simulink model "EcoSIM3_P2_C2"  (R2014b)
settings: Solver=ode1  SolverMode=SingleTasking  StartTime=0.0  StopTime=inf  FixedStep=0.01  RelTol=1e-3
PostLoadFcn:
  | %, if any(exist('dsrtsu_mdlpostloadfcn', 'file') == [2, 3, 6]), try dsrtsu_mdlpostloadfcn('Execute', bdroot); catch fprintf('Error in PostLoadFcn (dsrtsu_mdlpostloadfcn) for model "%s":\n %s\n', bdroot, lasterr); end, end,
InitFcn:
  | tic
  | %Startup_EcoSIM
values from neighbouring files (symbols this model uses):
  EngPwr = [0 5	10	15	20	25	30	35	40	45	50	55	60	65	70	75	80	85	90	95	100	105	110	115]    [Series_Maps.m]
  EngSpd = [0 477.4645 954.929 1909.858 2864.787 3819.716 4774.645 5729.574 6684.503]    [Series_Maps.m]
  EngTrq = [0	0	0	0	0	0	0	0	0	0	0	0	0	0	0	0	0	0	0	0	0	0	0	0 ... (first row only)    [Series_Maps.m]
  Power = [0 5 10 15 20 25 30]    [Series_Maps.m]
  Torque = [-50,-40,-30,-25,-20,-15,-10,-8,-6,-4,-2,0]    [Series_Maps.m]
undefined symbols (not defined in the file or in its folder): canChannel, Controls, DriveCycles, Driver, EM_EFF_MAP, EM_PwrLoss_MAP, Glbl, Plants, Veh_Dynamics
libraries: canmsglib x100, canlib x87, fl_lib x78, simulink x59, nesl_utility x40, sdl_lib x17, dspsigops x5, dspswit3 x3, dspstat3 x2, commnoisgen2 x1, dspfdesign x1
(part 15 of 15)

== stateflow chart EcoSIM3_P2_C2/Powertrain/BAS Motor/Soft ECU/Algorithm/BAS_Stateflow/BAS SoftECU ==
  note: Mode Request is similar to Inverter Enable / Disable
  state StartupShutdownSequence [group]
    state StartState
      during: Commanded_Torque = 0;
      %Loading EEPROM Parameters & carrying out POST (Power On Self Tests)
    state Standby
      % Entry point into Inverter
      % State Machine
    state Startup_Sequence
      state Inverter_Wait
        entry: FaultState=0;
        during: Commanded_Torque =0;
      state Inverter_Ready
        during: Commanded_Torque =0;
        entry: InverterStatusMode = 1;
        during: InverterStatusMode = 1;
      Inverter_Wait -> Inverter_Ready : [ModeRequest >= 1]
    state NormalOperation
      exit:Commanded_Torque=0;
      state Speed_Control_Mode
        state ValidSpeed
          entry: Commanded_Speed=Speed_Command;
          during: Commanded_Speed=Speed_Command;
        (default) -> StartupShutdownSequence.NormalOperation.Speed_Control_Mode.ValidSpeed
      state Torque_Control_Mode
        state SpeedGreaterThanMaxSpeed
          entry: Commanded_Torque=0;
          during: Commanded_Torque = 0;
        state ValidSpeed
          entry: Commanded_Torque=Torque_Command;
          during: Commanded_Torque=Torque_Command;
        state SpeedGreaterThanMaxSpeed1 [commented out]
          entry: Commanded_Torque=0;
        (default) -> (junction 53)
        (junction 53) -> SpeedGreaterThanMaxSpeed [order 1] : [abs (MotorSpeed) > MotorMaxSpeed]
        (junction 53) -> (junction 60) [order 2]
        SpeedGreaterThanMaxSpeed -> (junction 60) : [abs (MotorSpeed) <= MotorMaxSpeed]
        (junction 60) -> StartupShutdownSequence.NormalOperation.Torque_Control_Mode.ValidSpeed
        StartupShutdownSequence.NormalOperation.Torque_Control_Mode.ValidSpeed -> SpeedGreaterThanMaxSpeed [commented out] : [abs (MotorSpeed) > MotorMaxSpeed]
        StartupShutdownSequence.NormalOperation.Torque_Control_Mode.ValidSpeed -> SpeedGreaterThanMaxSpeed1 [commented out] : [MotorSpeed<= 83*BeltRatio]
        SpeedGreaterThanMaxSpeed1 -> StartupShutdownSequence.NormalOperation.Torque_Control_Mode.ValidSpeed [commented out] : [MotorSpeed>84*BeltRatio]
      (default) -> (junction 101)
      (junction 101) -> Speed_Control_Mode [order 2] : [ModeRequest == 2]
      (junction 101) -> Torque_Control_Mode [order 1] : [ModeRequest == 1]
    state ShutdownInProcess
    state FaultState
      entry: FaultState = 1;
      during: FaultState = 1;
      % to exit this state, power must be cycled
    (default) -> Standby
    Standby -> StartState : [Power_up == 1 && ...
        | POST_Fault == 0 ]
    StartState -> FaultState [order 2] : [Power_up == 1 ...
        | &&POST_Fault == 1]
    StartState -> Inverter_Wait [order 1] : [Power_up == 1 ...
        | &&POST_Fault == 0]
    ShutdownInProcess -> Standby : [Power_up == 0]
    (junction 28) -> ShutdownInProcess [order 2] : [Power_up ==0]
    FaultState -> ShutdownInProcess : [Power_up == 0 ]
    Inverter_Ready -> NormalOperation : [MotorFault==0]
    (junction 28) -> FaultState [order 1] : [MotorFault ==1]
    NormalOperation -> (junction 28) : [MotorFault==1]
  data: Power_up input; MotorFault input; ModeRequest input; Commanded_Torque output; MotorMaxSpeed input; POST_Fault input; InverterStatusMode output; Torque_Command input; MotorSpeed input; FaultState output; BeltRatio input; Commanded_Speed output; Speed_Command input

== stateflow chart EcoSIM3_P2_C2/Powertrain/Electric Motor /Soft ECU/Algorithm/Startup_Shutdown/Startup-Shutdown ==
  state StartupShutdownSequence [group]
    state StartState
      entry: VSM_Mode = 0;
      during: Commanded_Torque = 0;
      %Loading EEPROM Parameters & carrying out POST (Power On Self Tests)
    state Standby
      % Entry point into Inverter
      % State Machine
    state Startup_Sequence
      state Inverter_Wait
        entry: VSM_Mode = 4;
        during: VSM_Mode = 4;
        during: Commanded_Torque =0;
        % Precharge_Bypasseed_EEPROM = 1
      state InverterEnableLockout
        entry: VSM_Mode = 5;
        during: VSM_Mode = 5;
        during: Commanded_Torque =0;
        entry: Inverter_Enable_Lockout = 1;
        during:Inverter_Enable_Lockout = 1;
      state Wait
      state MotorReady
        entry: Inverter_Enable_Lockout = 0;
        entry: Inverter_Status=1;
        during: Inverter_Enable_Lockout = 0;
      state MotorOnCommand
        entry: VSM_Mode=6;
      Inverter_Wait -> InverterEnableLockout : [KeySwMode == 0 && ...
          | IgnitionKeySw == 2]
      InverterEnableLockout -> Wait : [Inverter_Enable == 0]
      Wait -> MotorReady : after(0.05,sec)
      MotorReady -> MotorOnCommand : [InternalMotorError==0 && Inverter_Enable == 1]
    state ShutdownInProcess
      entry: VSM_Mode = 14;
      entry: Inverter_Enable_Lockout=1;
      entry: Inverter_Status=0;
      during: VSM_Mode = 14;
    state FaultState
      entry: VSM_Mode = 7;
      during: VSM_Mode = 7;
    (junction 28) -> Standby [order 2]
    Standby -> StartState : [Power_up == 1]
    (default) -> (junction 28)
    ShutdownInProcess -> Standby : [KeySwMode == 0 && ...
        | IgnitionKeySw == 0 ...
        | && Power_up == 0]
    StartState -> FaultState [order 2] : [POST_Fault == 1]
    StartState -> Inverter_Wait [order 1] : [Power_up ==1 && ...
        | ~InternalMotorError && POST_Fault == 0 ...
        | && batt_mainc_stat == 1 ]
    (junction 28) -> FaultState [order 1] : [InternalMotorError ==1]
    FaultState -> ShutdownInProcess : [(KeySwMode == 0 && ...
        | IgnitionKeySw == 0) ]
    MotorOnCommand -> ShutdownInProcess [order 1] : [ShutdownRequest ==1]
    MotorOnCommand -> FaultState [order 2] : [RUN_Fault==1]
  data: Power_up input; VSM_Mode output; InternalMotorError input; batt_mainc_stat input; Inverter_Enable input; IgnitionKeySw input; Inverter_Enable_Lockout output; RUN_Fault input; Commanded_Torque local; ShutdownRequest input; KeySwMode input; POST_Fault input; Inverter_Status output

== stateflow chart EcoSIM3_P2_C2/Powertrain/Electric Motor /Soft ECU/Algorithm/Normal Operation/Normal_Operation ==
  state NormalOperation
    entry: set_direction=Rotation_Direction;
    entry: ShutdownRequest=0;
    exit: Commanded_Torque=0;
    state SpeedGreaterThanMaxSpeed
      entry: Commanded_Torque=0;
    state ValidSpeed
      entry: Commanded_Torque=Torque_Command;
      during: Commanded_Torque=Torque_Command;
    (default) -> (junction 9)
    (junction 9) -> SpeedGreaterThanMaxSpeed [order 1] : [abs (Motor_Speed) > Motor_MaxSpeed]
    (junction 9) -> (junction 10) [order 2]
    SpeedGreaterThanMaxSpeed -> (junction 10) : [abs (Motor_Speed) <= Motor_MaxSpeed]
    (junction 10) -> ValidSpeed
    ValidSpeed -> SpeedGreaterThanMaxSpeed : [abs (Motor_Speed) > Motor_MaxSpeed]
  state Fault
    entry: RUN_Fault=1;
  state ShutdownRequest
    entry: ShutdownRequest=1;
  (default) -> NormalOperation
  NormalOperation -> Fault [order 1] : [ InternalMotorError ==1||batt_mainc_stat==0]
  NormalOperation -> ShutdownRequest [order 2] : [IgnitionKeySw==0||...
      | Inverter_Enable==0]
  ShutdownRequest -> NormalOperation : [IgnitionKeySw==2||...
      | Inverter_Enable==1]
  data: Motor_Speed input; InternalMotorError input; Rotation_Direction input; set_direction local; Commanded_Torque output; Torque_Command input; batt_mainc_stat input; Inverter_Enable input; IgnitionKeySw input; RUN_Fault output; Motor_MaxSpeed input; ShutdownRequest output

== stateflow chart EcoSIM3_P2_C2/GCM/ProcessMode/Chart ==
  state Entry
    entry: charge_mode_request=0;
    Relay_Charge=0;
    Relay_Vehicle=0;
  state FaultModeDecideLater
  state VehicleRunMode
    entry: charge_mode_request=0;
    Relay_Charge=1;
    Relay_Vehicle=1;
  state ChargingMode
    entry: charge_mode_request=1;
    Relay_Charge=1;
    Relay_Vehicle=0;
  (default) -> Entry
  VehicleRunMode -> Entry : [Key_State==0]
  ChargingMode -> Entry [order 1] : [Key_State==0]
  Entry -> VehicleRunMode [order 1] : [Key_State==1 && ...
      | GCM_Wakeup_charge==0]
  Entry -> FaultModeDecideLater [order 3] : [Key_State==1 && ...
      | GCM_Wakeup_charge ==1]
  Entry -> ChargingMode [order 2] : [Key_State ==0 && ...
      | GCM_Wakeup_charge==1]
  ChargingMode -> FaultModeDecideLater [order 2] : [Key_State==1]
  data: Key_State input; GCM_Wakeup_charge input; charge_mode_request output; Relay_Charge output; Relay_Vehicle output

== matlab function EcoSIM3_P2_C2/Supervisory Controller/Functional Safety1/Functional Safety Algorithm/Fault Management/Truth Table ==
  data: u input; y output
function y = fcn(u)

aVarTruthTableCondition_1 = false;
aVarTruthTableCondition_2 = false;


% Example condition 1

aVarTruthTableCondition_1 = logical(u >= 0);

% Example condition 2

aVarTruthTableCondition_2 = logical(u ^ 2 <= 1);

if (aVarTruthTableCondition_1 && aVarTruthTableCondition_2)
    aFcnTruthTableAction_1();
elseif (~aVarTruthTableCondition_1 && ~aVarTruthTableCondition_2)
    aFcnTruthTableAction_1();
else % Default
    aFcnTruthTableAction_2();
end

function aFcnTruthTableAction_1()

% Example action 1 called from D1 & D2 column in condition table

y = u;

function aFcnTruthTableAction_2()

% Example action 2 called from D3 column in condition table

y = 1 / u;

== stateflow chart EcoSIM3_P2_C2/Powertrain/Engine/Soft ECU/Algorithm/ECM SoftECU ==
  state Entry
    entry: Torque_Cmd=0;
  state PoweredUp
    entry: Torque_Cmd=0;
  state PoweredUp1
    entry: Torque_Cmd=Torque_Request;
    du: Torque_Cmd=Torque_Request;
  state PoweredUp2
    entry: Torque_Cmd=0;
  (default) -> Entry
  PoweredUp1 -> Entry [order 1] : [ECM_Powerup==0]
  Entry -> PoweredUp : [ECM_Powerup==1]
  PoweredUp1 -> PoweredUp [order 2] : [PCM_Wake==0 || ...
      | ISP_R ==0]
  PoweredUp -> PoweredUp1 : [PCM_Wake==1 &&...
      | ISP_R==1]
  PoweredUp1 -> PoweredUp2 [order 3] : [Engine_Speed>Max_Speed]
  PoweredUp2 -> PoweredUp1 : [Engine_Speed <(Max_Speed-10)]
  data: Engine_Speed input; ECM_Powerup input; Torque_Cmd output; Torque_Request input; PCM_Wake input; ISP_R input; Max_Speed input

== stateflow chart EcoSIM3_P2_C2/Supervisory Controller/Mode Operation/Limited EV/Temperature Limiting/Chart ==
  state EM
    entry: out=1
  state Normal
    entry: out=4;
  state Inverter
    entry: out=2
  state Battery
    entry: out=3
  Normal -> EM [order 1] : [EM>100]
  (default) -> Normal
  Normal -> Inverter [order 2] : [Inverter>70]
  Normal -> Battery [order 3] : [Battery>50]
  data: EM input; Inverter input; Battery input; out output

== stateflow chart EcoSIM3_P2_C2/Fault Insertion/ESS Triggers/Chart ==
  state init
    en: output = 40;
  state stage1
    en: output = 56;
  state stage2
    en: output = 66;
  state stage3
    en: output = 40;
  (default) -> init
  init -> stage1 : [in == 1]
  stage1 -> stage2 : after(20, sec)
  stage2 -> stage3 : after(20, sec)
  data: in input; output output

== stateflow chart EcoSIM3_P2_C2/Supervisory Controller/Mode Operation/Shutdown/EM Handshake ==
  state Entry
  state DisableInverter
    entry: Inverter_Enable=0;
    during: Inverter_Enable=0;
  (default) -> Entry
  Entry -> DisableInverter : [Inverter_Enable_Lockout==1]
  data: Inverter_Enable_Lockout input; Inverter_Enable output

== stateflow chart EcoSIM3_P2_C2/Supervisory Controller/Mode Operation/Shutdown/Shutdown/ESS Handshake ==
  note: The ESS handshake ensures that the hsc_bcm_enable signal commands is sent by the supervisory only when the bcm is in the appropriate readiness state
  state WaitforBCMReady1
  state Disable
    entry: hsc_bcm_enable=0;
    during: hsc_bcm_enable=0;
  state OpenContactors
    entry:hsc_bcm_mainc_close=0;
    entry: hsc_bcm_leakage_ena=1;
    during:hsc_bcm_mainc_close=0;
    during:hsc_bcm_enable=0;
  Disable -> WaitforBCMReady1 : [bcm_ready==0]
  OpenContactors -> Disable : [bcm_mainc_stat==0]
  (default) -> OpenContactors
  data: bcm_ready input double; bcm_cpwr_cmd input double; bcm_cpwr_mon input double; hsc_bcm_enable output double; hsc_bcm_mainc_close output double; hsc_bcm_leakage_ena output; bcm_veh_mon input; Veh_Start input double; bcm_mainc_stat input

== stateflow chart EcoSIM3_P2_C2/Supervisory Controller/Mode Operation/Startup/BAS Start up/BAS Handshake ==
  state Entry
    entry: BAS_Mode_Request=0;
  state EnableBASInverter
    entry: BAS_Mode_Request=1;
  (default) -> Entry
  Entry -> EnableBASInverter : [BAS_Fault_Status==0 ...
      | && bcm_mainc_stat==1]
  data: BAS_Fault_Status input; bcm_mainc_stat input; BAS_Mode_Request output

== stateflow chart EcoSIM3_P2_C2/Supervisory Controller/Mode Operation/Startup/Battery Start Up /ESS Handshake ==
  note: The ESS handshake ensures that the hsc_bcm_enable signal commands is sent by the supervisory only when the bcm is in the appropriate readiness state
  state Entry
    entry: hsc_bcm_enable=0;
    en: hsc_bcm_leakage_ena=1;
    en: hsc_bcm_mainc_close=0;
  state WaitforBCMReady
  state Enable
    entry: hsc_bcm_enable=1;
    during: hsc_bcm_enable=1;
  state CloseContactors
    entry:hsc_bcm_mainc_close=1;
    during:hsc_bcm_mainc_close=1;
    during:hsc_bcm_enable=1;
  (default) -> Entry
  Entry -> WaitforBCMReady : [bcm_veh_mon==1 && Veh_Start==1]
  WaitforBCMReady -> Enable : [bcm_ready==1]
  Enable -> CloseContactors : [bcm_cpwr_cmd==1 && bcm_cpwr_mon==1]
  data: bcm_ready input double; bcm_cpwr_cmd input double; bcm_cpwr_mon input double; hsc_bcm_enable output double; hsc_bcm_mainc_close output double; hsc_bcm_leakage_ena output; bcm_veh_mon input; bcm_mainc_stat input; Veh_Start input double

== stateflow chart EcoSIM3_P2_C2/Supervisory Controller/Mode Operation/Startup/EM Start up/EM Handshake ==
  state Entry
  state DisableInverter
    entry: Inverter_Enable=0;
    during: Inverter_Enable=0;
  state EnableInverter
    entry: Inverter_Enable=1;
    during: Inverter_Enable=1;
  (default) -> Entry
  Entry -> DisableInverter : [Inverter_Enable_Lockout==1]
  EnableInverter -> DisableInverter : [Inverter_Enable_Lockout==1]
  DisableInverter -> EnableInverter : [Inverter_Enable_Lockout==0 ...
      | && bcm_mainc_stat==1]
  data: bcm_mainc_stat input; Inverter_Enable_Lockout input; Inverter_Enable output

== stateflow chart EcoSIM3_P2_C2/Supervisory Controller/Mode Operation/Startup/Vehicle Ready ==
  state Entry
    entry: Vehicle_Ready=0;
  state Started
    entry:Vehicle_Ready=1;
  (default) -> Entry
  Entry -> Started : [bcm_mainc_stat==1 ...
      | && Inverter_Enable ==1 ...
      | && BAS_Mode_Request ==1 ...
      | &&Startup_Complete==1]
  data: Startup_Complete input; bcm_mainc_stat input; Inverter_Enable input; BAS_Mode_Request input; Vehicle_Ready output

== stateflow chart EcoSIM3_P2_C2/Supervisory Controller/Mode Selection /Limp Home Mode Selection  /Chart ==
  state Engine_Only
    entry: VEH_Mode=3;
  state EV_Limited
    entry: VEH_Mode=5;
  state Normal_Operation
    entry: VEH_Mode=2;
  state Shutdown
    entry: VEH_Mode=6;
  Normal_Operation -> Engine_Only [order 1] : [Fault_Code==1]
  Engine_Only -> Shutdown : [Fault_Code==3]
  Normal_Operation -> EV_Limited [order 2] : [Fault_Code==2]
  EV_Limited -> Shutdown : [Fault_Code==3]
  Normal_Operation -> Shutdown [order 3] : [Fault_Code==3]
  (default) -> (junction 7)
  (junction 7) -> Normal_Operation : [Fault_Code==0]
  data: VEH_Mode output; Fault_Code input

== stateflow chart EcoSIM3_P2_C2/Supervisory Controller/Mode Selection /Mode Selection  ==
  state Vehicle_On
    state Series
      entry: VEH_Mode=9;
    state CD_Normal
      entry: VEH_Mode=2;
    state Engine_on
      entry: VEH_Mode=3;
    state Engine_Start
      entry: VEH_Mode=4;
    Engine_on -> CD_Normal : [eng_switch==0&&SOC<Min_SOC]
    Series -> CD_Normal : [cs_switch==0||SOC>95]
    Engine_Start -> Series [order 2] : [eng_on==1&&...
        | cs_switch==1]
    (default) -> CD_Normal
    Engine_Start -> Engine_on [order 1] : [eng_on==1&&...
        | eng_switch==1]
    CD_Normal -> Engine_Start : [SOC<Min_SOC || eng_switch==1||...
        | cs_switch==1]
  state Startup
    entry: VEH_Mode=1;
  state Accessory
    entry: VEH_Mode=7;
  state Shutdown
    entry: VEH_Mode=6;
  state Charging
    entry: VEH_Mode=8;
  (default) -> Startup
  Startup -> Vehicle_On [order 1] : [Key_State==2&&Vehicle_Ready>0]
  Startup -> Charging [order 3] : [bcm_on_plug==1]
  Shutdown -> Startup : [Shutdown_Complete==1&&Key_State>0]
  Startup -> Accessory [order 2] : [Key_State==1]
  Vehicle_On -> Accessory [order 2] : [Key_State==1]
  Vehicle_On -> Charging [order 3] : [bcm_on_plug==1]
  Vehicle_On -> Shutdown [order 1] : [Key_State==0]
  Accessory -> Shutdown : [Key_State==0]
  Charging -> Shutdown : [bcm_on_plug==0]
  data: Veh_Spd input; SOC input; VEH_Mode output; Min_SOC input; beta input; Key_State input; eng_on input; eng_switch input; cs_switch input; Vehicle_Ready input; Shutdown_Complete input; bcm_on_plug input

== matlab function EcoSIM3_P2_C2/Supervisory Controller/PRNDL/Determine Gear/Truth Table ==
  data: y output; PRNDL input double; Force_Neutral input boolean; Force_Park input boolean
function y = fcn(PRNDL, Force_Neutral, Force_Park)

aVarTruthTableCondition_1 = false;
aVarTruthTableCondition_2 = false;
aVarTruthTableCondition_3 = false;
aVarTruthTableCondition_4 = false;
aVarTruthTableCondition_5 = false;
aVarTruthTableCondition_6 = false;


% Force Park

aVarTruthTableCondition_1 = logical(Force_Park == 1);

% Force Neutral

aVarTruthTableCondition_2 = logical(Force_Neutral == 1);

% PRNDL set to P

aVarTruthTableCondition_3 = logical(PRNDL == 1);

% PRNDL set to R

aVarTruthTableCondition_4 = logical(PRNDL == 2);

% PRNDL set to N

aVarTruthTableCondition_5 = logical(PRNDL == 3);

% PRNDL set to D

aVarTruthTableCondition_6 = logical(PRNDL == 4);

if (aVarTruthTableCondition_1)
    aFcnTruthTableAction_1();
elseif (aVarTruthTableCondition_2)
    aFcnTruthTableAction_3();
elseif (aVarTruthTableCondition_3)
    aFcnTruthTableAction_1();
elseif (~aVarTruthTableCondition_1 && ~aVarTruthTableCondition_2 && ~aVarTruthTableCondition_3 && aVarTruthTableCondition_4 && ~aVarTruthTableCondition_5 && ~aVarTruthTableCondition_6)
    aFcnTruthTableAction_2();
elseif (~aVarTruthTableCondition_1 && ~aVarTruthTableCondition_3 && ~aVarTruthTableCondition_4 && aVarTruthTableCondition_5 && ~aVarTruthTableCondition_6)
    aFcnTruthTableAction_3();
elseif (~aVarTruthTableCondition_1 && ~aVarTruthTableCondition_2 && ~aVarTruthTableCondition_3 && ~aVarTruthTableCondition_4 && ~aVarTruthTableCondition_5 && aVarTruthTableCondition_6)
    aFcnTruthTableAction_4();
else % Default
    aFcnTruthTableAction_1();
end

function aFcnTruthTableAction_1()

% Vehicle is in PARK gear

y = 1;

function aFcnTruthTableAction_2()

% Vehicle is in REVERSE gear

y = 2;

function aFcnTruthTableAction_3()

% Vehicle is in NEUTRAL gear

y = 3;

function aFcnTruthTableAction_4()

% Vehicle is in DRIVE gear

y = 4;

== stateflow chart EcoSIM3_P2_C2/Supervisory Controller/Simple Fault Detection/Fault Code Determination ==
  state Normal_Operation
    entry: Fault_Code=0;
  state Limited_EV
    entry: Fault_Code=2;
  state Shutdown
    entry: Fault_Code=3;
  Limited_EV -> Normal_Operation [order 2] : [EM_Temp<EM_Warning-3&&...
      | Inverter_Temp<Inverter_Warning-3&&...
      | Battery_Temp<Battery_Warning-3]
  Normal_Operation -> Limited_EV [order 1] : [EM_Temp>EM_Warning&&EM_Temp<EM_Shutdown||...
      | Inverter_Temp>Inverter_Warning&&Inverter_Temp<Inverter_Shutdown||...
      | Battery_Temp>Battery_Warning&&Battery_Temp<Battery_Shutdown]
  (default) -> Normal_Operation
  Limited_EV -> Shutdown [order 1] : [EM_Temp>=EM_Shutdown||...
      | Inverter_Temp>=Inverter_Shutdown||...
      | Battery_Temp>=Battery_Shutdown]
  Normal_Operation -> Shutdown [order 2] : [EM_Temp>=EM_Shutdown||...
      | Inverter_Temp>=Inverter_Shutdown||...
      | Battery_Temp>=Battery_Shutdown]
  data: EM_Temp input; Battery_Temp input; Inverter_Temp input; Fault_Code output; EM_Warning input; EM_Shutdown input; Inverter_Warning input; Inverter_Shutdown input; Battery_Warning input; Battery_Shutdown input

== matlab function EcoSIM3_P2_C2/Supervisory Controller/PRNDL/Determine Gear1/Truth Table ==
  data: y output; PRNDL input double; Force_Neutral input boolean
function y = fcn(PRNDL, Force_Neutral)

aVarTruthTableCondition_1 = false;
aVarTruthTableCondition_2 = false;
aVarTruthTableCondition_3 = false;
aVarTruthTableCondition_4 = false;
aVarTruthTableCondition_5 = false;
aVarTruthTableCondition_6 = false;


% Force Neutral

aVarTruthTableCondition_1 = logical(Force_Neutral == 1);

% PRNDL invalid gear

aVarTruthTableCondition_2 = logical(PRNDL == 0);

% PRNDL set to P

aVarTruthTableCondition_3 = logical(PRNDL == 1);

% PRNDL set to R

aVarTruthTableCondition_4 = logical(PRNDL == 2);

% PRNDL set to N

aVarTruthTableCondition_5 = logical(PRNDL == 3);

% PRNDL set to D

aVarTruthTableCondition_6 = logical(PRNDL == 4);

if (aVarTruthTableCondition_1)
    aFcnTruthTableAction_3();
elseif (aVarTruthTableCondition_2)
    aFcnTruthTableAction_3();
elseif (~aVarTruthTableCondition_1 && ~aVarTruthTableCondition_2 && ~aVarTruthTableCondition_3 && aVarTruthTableCondition_4 && ~aVarTruthTableCondition_5 && ~aVarTruthTableCondition_6)
    aFcnTruthTableAction_2();
elseif (~aVarTruthTableCondition_1 && ~aVarTruthTableCondition_2 && ~aVarTruthTableCondition_3 && ~aVarTruthTableCondition_4 && ~aVarTruthTableCondition_5 && aVarTruthTableCondition_6)
    aFcnTruthTableAction_1();
else % Default
    aFcnTruthTableAction_3();
end

function aFcnTruthTableAction_1()

% Vehicle is in FORWARD gear

y = 1;

function aFcnTruthTableAction_2()

% Vehicle is in REVERSE gear

y = 2;

function aFcnTruthTableAction_3()

% Vehicle is in NEUTRAL gear

y = 3;
